simulink model "Waehrungsmodelle"  (R2014a)
settings: Solver=ode1  StartTime=0.0  StopTime=100  FixedStep=1  MaxStep=1  MinStep=1  RelTol=1e-3
(part 1 of 18)
settings Model: Creator=christoph  LastModifiedBy=christoph

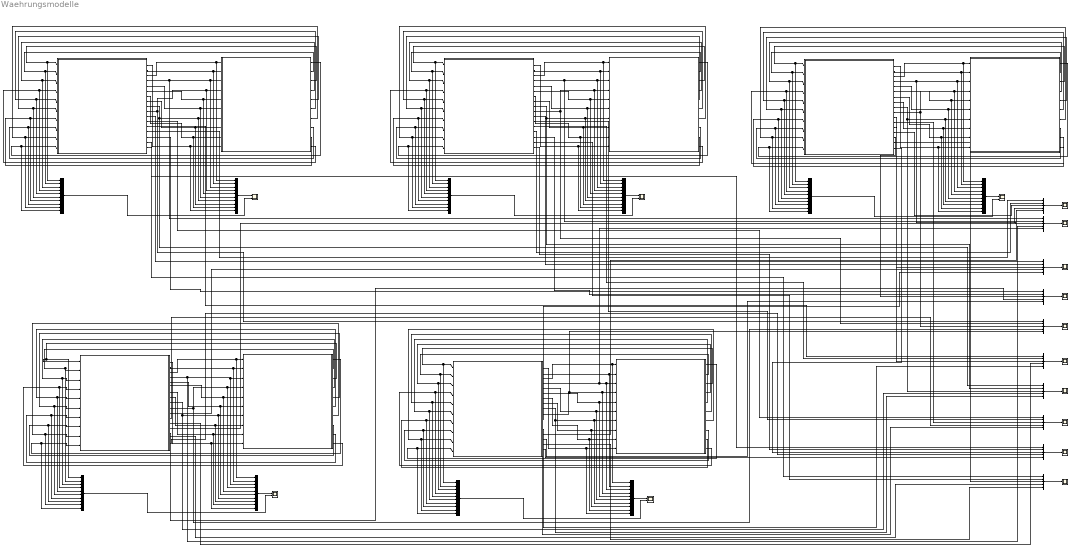
== system Waehrungsmodelle ==
  note: Ungedecktes Währungsmodell
  note: Freies Geld Währungsmodell
  note: Fliessendes Geld Währungsmodell
  note: Vollgeld Währungsmodell
  note: Gedecktes Währungsmodell
  Arbeitslohn : Scope
      settings: ShowLegends=on  YMin=0  YMax=70  SaveName=ScopeData25
  Arbeitslosigkeit : Scope
      settings: ShowLegends=on  YMin=-0.1  YMax=1  SaveName=ScopeData22
  Bankenzins : Scope
      settings: ShowLegends=on  YMin=-0.2  YMax=0.6  SaveName=ScopeData20
  Fließendes Währungssystem : Subsystem
  Freies Geld Währungssystem : Subsystem
  Gedecktes Währungssystem : Subsystem
  Gesamtkredite : Scope
      settings: ShowLegends=on  YMin=0  YMax=9000  SaveName=ScopeData23
  Güterpreise : Scope
      settings: TickLabels=on  ShowLegends=on  TimeRange=100  YMin=0  YMax=35  SaveName=ScopeData21
  Inflation (Preisstabilität) : Scope
      settings: ShowLegends=on  YMin=-0.1  YMax=0.2  SaveName=ScopeData18
  Konsum Ausland : Scope
      settings: ShowLegends=on  YMin=-0.1  YMax=0.2  SaveName=ScopeData27
  Konsum Inland : Scope
      settings: ShowLegends=on  YMin=-0.1  YMax=0.2  SaveName=ScopeData26
  Mux{,1..9} (10 alike) : Mux  Inputs=10
  Mux{10..19} (10 alike) : Mux  Inputs=5
  Notenbankgeldmange / Maximale Geldmenge : Scope
      settings: ShowLegends=on  YMin=0  YMax=10000  SaveName=ScopeData19
  Notenbankzins : Scope
      settings: ShowLegends=on  YMin=-0.05  YMax=0.15  SaveName=ScopeData24
  Scope{,1..4} (5 alike) : Scope  NumInputPorts=2
      Scope settings: ShowLegends=on  YMin=-100~-100  YMax=900~900  SaveName=ScopeData8
      Scope1 settings: ShowLegends=on  YMin=-100~-100  YMax=900~900  SaveName=ScopeData15
      Scope2 settings: ShowLegends=on  YMin=-100~-100  YMax=900~900  SaveName=ScopeData13
      Scope3 settings: ShowLegends=on  YMin=-100~-100  YMax=900~900  SaveName=ScopeData16
      Scope4 settings: ShowLegends=on  YMin=-100~-100  YMax=900~900  SaveName=ScopeData17
  Vollgeld Währungssystem : Subsystem
  Währungssystem1 : Subsystem
  Währungssystem2 : Subsystem
  Währungssystem3 : Subsystem
  Währungssystem4 : Subsystem
  Währungssystem5 : Subsystem
  Währungssystem6 : Subsystem
  wires:
  Währungssystem1/2(Kreditbedarf Ausland Unternehmen) -> Währungssystem2/2(Kreditbedarf der Unternehmen im Ausland), Mux/2
  Währungssystem1/3(Kreditbedarf Ausland Haushalte) -> Währungssystem2/1(Kreditbedarf der Haushalte im Ausland), Mux/1
  Währungssystem1/1(Güterangebot an  Ausland) -> Währungssystem2/10(Güterangebot vom  Ausland), Mux/10
  Währungssystem1/5(Bank: Kreditrückzahlung der Unternemen Ausland) -> Währungssystem2/6(Kreditrückzahlung der Unternehmen Ausland), Mux/6
  Währungssystem1/6("Bank: Kreditvergabe der Unternemen Ausland ") -> Währungssystem2/5(Neue Kreditvergabe der Unternehmen Ausland), Mux/5
  Währungssystem1/7(Bank: Kreditrückzahlung der Haushalte Ausland) -> Währungssystem2/9(Kreditrückzahlung der Haushalte Ausland), Mux/9
  Währungssystem1/8("Bank: Kreditvergabe der Haushalte Ausland ") -> Währungssystem2/8(Neue Kreditvergabe der Haushalte Ausland), Mux/8
  Währungssystem2/1(Güterangebot an  Ausland) -> Mux1/10, Währungssystem1/10(Güterangebot vom  Ausland)
  Währungssystem2/2(Kreditbedarf Ausland Unternehmen) -> Mux1/2, Währungssystem1/2(Kreditbedarf der Unternehmen im Ausland)
  Währungssystem2/3(Kreditbedarf Ausland Haushalte) -> Mux1/1, Währungssystem1/1(Kreditbedarf der Haushalte im Ausland)
  Währungssystem2/4(Güterkonsum vom Ausland) -> Mux1/3, Währungssystem1/3(Güterkonsum Ausland)
  Währungssystem2/5(Bank: Kreditrückzahlung der Unternemen Ausland) -> Mux1/6, Währungssystem1/6(Kreditrückzahlung der Unternehmen Ausland)
  Währungssystem2/6("Bank: Kreditvergabe der Unternemen Ausland ") -> Mux1/5, Währungssystem1/5(Neue Kreditvergabe der Unternehmen Ausland)
  Währungssystem2/7(Bank: Kreditrückzahlung der Haushalte Ausland) -> Mux1/9, Währungssystem1/9(Kreditrückzahlung der Haushalte Ausland)
  Währungssystem2/8("Bank: Kreditvergabe der Haushalte Ausland ") -> Mux1/8, Währungssystem1/8(Neue Kreditvergabe der Haushalte Ausland)
  Währungssystem2/9(Güterpreis) -> Mux1/7, Währungssystem1/7(Güterpreis Ausland)
  Währungssystem2/10(Bankenzinssatz) -> Mux1/4, Währungssystem1/4(Zinssatz Ausland)
  Mux/1 -> Scope/1
  Mux1/1 -> Scope/2
  Freies Geld Währungssystem/2(Kreditbedarf Ausland Unternehmen) -> Währungssystem4/2(Kreditbedarf der Unternehmen im Ausland), Mux2/2
  Freies Geld Währungssystem/3(Kreditbedarf Ausland Haushalte) -> Währungssystem4/1(Kreditbedarf der Haushalte im Ausland), Mux2/1
  Freies Geld Währungssystem/4(Güterkonsum vom Ausland) -> Mux19/4, Währungssystem4/3(Güterkonsum Ausland), Mux2/3
  Freies Geld Währungssystem/1(Güterangebot an  Ausland) -> Währungssystem4/10(Güterangebot vom  Ausland), Mux2/10
  Freies Geld Währungssystem/5(Bank: Kreditrückzahlung der Unternemen Ausland) -> Währungssystem4/6(Kreditrückzahlung der Unternehmen Ausland), Mux2/6
  Freies Geld Währungssystem/6("Bank: Kreditvergabe der Unternemen Ausland ") -> Währungssystem4/5(Neue Kreditvergabe der Unternehmen Ausland), Mux2/5
  Freies Geld Währungssystem/7(Bank: Kreditrückzahlung der Haushalte Ausland) -> Währungssystem4/9(Kreditrückzahlung der Haushalte Ausland), Mux2/9
  Freies Geld Währungssystem/8("Bank: Kreditvergabe der Haushalte Ausland ") -> Währungssystem4/8(Neue Kreditvergabe der Haushalte Ausland), Mux2/8
  Währungssystem4/1(Güterangebot an  Ausland) -> Mux3/10, Freies Geld Währungssystem/10(Güterangebot vom  Ausland)
  Währungssystem4/2(Kreditbedarf Ausland Unternehmen) -> Mux3/2, Freies Geld Währungssystem/2(Kreditbedarf der Unternehmen im Ausland)
  Währungssystem4/3(Kreditbedarf Ausland Haushalte) -> Mux3/1, Freies Geld Währungssystem/1(Kreditbedarf der Haushalte im Ausland)
  Währungssystem4/4(Güterkonsum vom Ausland) -> Mux3/3, Freies Geld Währungssystem/3(Güterkonsum Ausland)
  Währungssystem4/5(Bank: Kreditrückzahlung der Unternemen Ausland) -> Mux3/6, Freies Geld Währungssystem/6(Kreditrückzahlung der Unternehmen Ausland)
  Währungssystem4/6("Bank: Kreditvergabe der Unternemen Ausland ") -> Mux3/5, Freies Geld Währungssystem/5(Neue Kreditvergabe der Unternehmen Ausland)
  Währungssystem4/7(Bank: Kreditrückzahlung der Haushalte Ausland) -> Mux3/9, Freies Geld Währungssystem/9(Kreditrückzahlung der Haushalte Ausland)
  Währungssystem4/8("Bank: Kreditvergabe der Haushalte Ausland ") -> Mux3/8, Freies Geld Währungssystem/8(Neue Kreditvergabe der Haushalte Ausland)
  Währungssystem4/9(Güterpreis) -> Mux3/7, Freies Geld Währungssystem/7(Güterpreis Ausland)
  Währungssystem4/10(Bankenzinssatz) -> Mux3/4, Freies Geld Währungssystem/4(Zinssatz Ausland)
  Mux2/1 -> Scope1/1
  Mux3/1 -> Scope1/2
  Fließendes Währungssystem/2(Kreditbedarf Ausland Unternehmen) -> Währungssystem5/2(Kreditbedarf der Unternehmen im Ausland), Mux4/2
  Fließendes Währungssystem/3(Kreditbedarf Ausland Haushalte) -> Währungssystem5/1(Kreditbedarf der Haushalte im Ausland), Mux4/1
  Fließendes Währungssystem/4(Güterkonsum vom Ausland) -> Mux19/5, Währungssystem5/3(Güterkonsum Ausland), Mux4/3
  Fließendes Währungssystem/1(Güterangebot an  Ausland) -> Währungssystem5/10(Güterangebot vom  Ausland), Mux4/10
  Fließendes Währungssystem/5(Bank: Kreditrückzahlung der Unternemen Ausland) -> Währungssystem5/6(Kreditrückzahlung der Unternehmen Ausland), Mux4/6
  Fließendes Währungssystem/6("Bank: Kreditvergabe der Unternemen Ausland ") -> Währungssystem5/5(Neue Kreditvergabe der Unternehmen Ausland), Mux4/5
  Fließendes Währungssystem/7(Bank: Kreditrückzahlung der Haushalte Ausland) -> Währungssystem5/9(Kreditrückzahlung der Haushalte Ausland), Mux4/9
  Fließendes Währungssystem/8("Bank: Kreditvergabe der Haushalte Ausland ") -> Währungssystem5/8(Neue Kreditvergabe der Haushalte Ausland), Mux4/8
  Währungssystem5/1(Güterangebot an  Ausland) -> Mux5/10, Fließendes Währungssystem/10(Güterangebot vom  Ausland)
  Währungssystem5/2(Kreditbedarf Ausland Unternehmen) -> Mux5/2, Fließendes Währungssystem/2(Kreditbedarf der Unternehmen im Ausland)
  Währungssystem5/3(Kreditbedarf Ausland Haushalte) -> Mux5/1, Fließendes Währungssystem/1(Kreditbedarf der Haushalte im Ausland)
  Währungssystem5/4(Güterkonsum vom Ausland) -> Mux5/3, Fließendes Währungssystem/3(Güterkonsum Ausland)
  Währungssystem5/5(Bank: Kreditrückzahlung der Unternemen Ausland) -> Mux5/6, Fließendes Währungssystem/6(Kreditrückzahlung der Unternehmen Ausland)
  Währungssystem5/6("Bank: Kreditvergabe der Unternemen Ausland ") -> Mux5/5, Fließendes Währungssystem/5(Neue Kreditvergabe der Unternehmen Ausland)
  Währungssystem5/7(Bank: Kreditrückzahlung der Haushalte Ausland) -> Mux5/9, Fließendes Währungssystem/9(Kreditrückzahlung der Haushalte Ausland)
  Währungssystem5/8("Bank: Kreditvergabe der Haushalte Ausland ") -> Mux5/8, Fließendes Währungssystem/8(Neue Kreditvergabe der Haushalte Ausland)
  Währungssystem5/9(Güterpreis) -> Mux5/7, Fließendes Währungssystem/7(Güterpreis Ausland)
  Währungssystem5/10(Bankenzinssatz) -> Mux5/4, Fließendes Währungssystem/4(Zinssatz Ausland)
  Mux4/1 -> Scope2/1
  Mux5/1 -> Scope2/2
  Vollgeld Währungssystem/2(Kreditbedarf Ausland Unternehmen) -> Währungssystem3/2(Kreditbedarf der Unternehmen im Ausland), Mux6/2
  Vollgeld Währungssystem/3(Kreditbedarf Ausland Haushalte) -> Währungssystem3/1(Kreditbedarf der Haushalte im Ausland), Mux6/1
  Vollgeld Währungssystem/4(Güterkonsum vom Ausland) -> Mux19/2, Währungssystem3/3(Güterkonsum Ausland), Mux6/3
  Vollgeld Währungssystem/1(Güterangebot an  Ausland) -> Währungssystem3/10(Güterangebot vom  Ausland), Mux6/10
  Vollgeld Währungssystem/5(Bank: Kreditrückzahlung der Unternemen Ausland) -> Währungssystem3/6(Kreditrückzahlung der Unternehmen Ausland), Mux6/6
  Vollgeld Währungssystem/6("Bank: Kreditvergabe der Unternemen Ausland ") -> Währungssystem3/5(Neue Kreditvergabe der Unternehmen Ausland), Mux6/5
  Vollgeld Währungssystem/7(Bank: Kreditrückzahlung der Haushalte Ausland) -> Währungssystem3/9(Kreditrückzahlung der Haushalte Ausland), Mux6/9
  Vollgeld Währungssystem/8("Bank: Kreditvergabe der Haushalte Ausland ") -> Währungssystem3/8(Neue Kreditvergabe der Haushalte Ausland), Mux6/8
  Vollgeld Währungssystem/9(Güterpreis) -> Währungssystem3/7(Güterpreis Ausland), Mux6/7, Mux14/2
  Währungssystem3/1(Güterangebot an  Ausland) -> Mux7/10, Vollgeld Währungssystem/10(Güterangebot vom  Ausland)
  Währungssystem3/2(Kreditbedarf Ausland Unternehmen) -> Mux7/2, Vollgeld Währungssystem/2(Kreditbedarf der Unternehmen im Ausland)
  Währungssystem3/3(Kreditbedarf Ausland Haushalte) -> Mux7/1, Vollgeld Währungssystem/1(Kreditbedarf der Haushalte im Ausland)
  Währungssystem3/4(Güterkonsum vom Ausland) -> Mux7/3, Vollgeld Währungssystem/3(Güterkonsum Ausland)
  Währungssystem3/5(Bank: Kreditrückzahlung der Unternemen Ausland) -> Mux7/6, Vollgeld Währungssystem/6(Kreditrückzahlung der Unternehmen Ausland)
  Währungssystem3/6("Bank: Kreditvergabe der Unternemen Ausland ") -> Mux7/5, Vollgeld Währungssystem/5(Neue Kreditvergabe der Unternehmen Ausland)
  Währungssystem3/7(Bank: Kreditrückzahlung der Haushalte Ausland) -> Mux7/9, Vollgeld Währungssystem/9(Kreditrückzahlung der Haushalte Ausland)
  Währungssystem3/8("Bank: Kreditvergabe der Haushalte Ausland ") -> Mux7/8, Vollgeld Währungssystem/8(Neue Kreditvergabe der Haushalte Ausland)
  Währungssystem3/9(Güterpreis) -> Mux7/7, Vollgeld Währungssystem/7(Güterpreis Ausland)
  Währungssystem3/10(Bankenzinssatz) -> Mux7/4, Vollgeld Währungssystem/4(Zinssatz Ausland)
  Mux6/1 -> Scope3/1
  Mux7/1 -> Scope3/2
  Gedecktes Währungssystem/2(Kreditbedarf Ausland Unternehmen) -> Währungssystem6/2(Kreditbedarf der Unternehmen im Ausland), Mux8/2
  Gedecktes Währungssystem/3(Kreditbedarf Ausland Haushalte) -> Währungssystem6/1(Kreditbedarf der Haushalte im Ausland), Mux8/1
  Gedecktes Währungssystem/4(Güterkonsum vom Ausland) -> Mux19/3, Währungssystem6/3(Güterkonsum Ausland), Mux8/3
  Gedecktes Währungssystem/1(Güterangebot an  Ausland) -> Währungssystem6/10(Güterangebot vom  Ausland), Mux8/10
  Gedecktes Währungssystem/5(Bank: Kreditrückzahlung der Unternemen Ausland) -> Währungssystem6/6(Kreditrückzahlung der Unternehmen Ausland), Mux8/6
  Gedecktes Währungssystem/6("Bank: Kreditvergabe der Unternemen Ausland ") -> Währungssystem6/5(Neue Kreditvergabe der Unternehmen Ausland), Mux8/5
  Gedecktes Währungssystem/7(Bank: Kreditrückzahlung der Haushalte Ausland) -> Währungssystem6/9(Kreditrückzahlung der Haushalte Ausland), Mux8/9
  Gedecktes Währungssystem/8("Bank: Kreditvergabe der Haushalte Ausland ") -> Währungssystem6/8(Neue Kreditvergabe der Haushalte Ausland), Mux8/8
  Gedecktes Währungssystem/9(Güterpreis) -> Mux14/3, Währungssystem6/7(Güterpreis Ausland), Mux8/7
  Währungssystem6/1(Güterangebot an  Ausland) -> Mux9/10, Gedecktes Währungssystem/10(Güterangebot vom  Ausland)
  Währungssystem6/2(Kreditbedarf Ausland Unternehmen) -> Mux9/2, Gedecktes Währungssystem/2(Kreditbedarf der Unternehmen im Ausland)
  Währungssystem6/3(Kreditbedarf Ausland Haushalte) -> Mux9/1, Gedecktes Währungssystem/1(Kreditbedarf der Haushalte im Ausland)
  Währungssystem6/4(Güterkonsum vom Ausland) -> Mux9/3, Gedecktes Währungssystem/3(Güterkonsum Ausland)
  Währungssystem6/5(Bank: Kreditrückzahlung der Unternemen Ausland) -> Mux9/6, Gedecktes Währungssystem/6(Kreditrückzahlung der Unternehmen Ausland)
  Währungssystem6/6("Bank: Kreditvergabe der Unternemen Ausland ") -> Mux9/5, Gedecktes Währungssystem/5(Neue Kreditvergabe der Unternehmen Ausland)
  Währungssystem6/7(Bank: Kreditrückzahlung der Haushalte Ausland) -> Mux9/9, Gedecktes Währungssystem/9(Kreditrückzahlung der Haushalte Ausland)
  Währungssystem6/8("Bank: Kreditvergabe der Haushalte Ausland ") -> Mux9/8, Gedecktes Währungssystem/8(Neue Kreditvergabe der Haushalte Ausland)
  Währungssystem6/9(Güterpreis) -> Mux9/7, Gedecktes Währungssystem/7(Güterpreis Ausland)
  Währungssystem6/10(Bankenzinssatz) -> Mux9/4, Gedecktes Währungssystem/4(Zinssatz Ausland)
  Mux8/1 -> Scope4/1
  Mux9/1 -> Scope4/2
  Mux10/1 -> Inflation (Preisstabilität)/1
  Gedecktes Währungssystem/11(Inflation) -> Mux10/3
  Vollgeld Währungssystem/11(Inflation) -> Mux10/2
  Währungssystem1/11(Inflation) -> Mux10/1
  Freies Geld Währungssystem/11(Inflation) -> Mux10/4
  Fließendes Währungssystem/11(Inflation) -> Mux10/5
  Mux11/1 -> Notenbankgeldmange / Maximale Geldmenge/1
  Gedecktes Währungssystem/15(Notenbankgeldmenge) -> Mux11/3
  Währungssystem1/15(Notenbankgeldmenge) -> Mux11/1
  Vollgeld Währungssystem/15(Notenbankgeldmenge) -> Mux11/2
  Freies Geld Währungssystem/15(Maximale Geldmenge) -> Mux11/4
  Fließendes Währungssystem/15(Notenbankgeldmenge) -> Mux11/5
  Mux12/1 -> Bankenzins/1
  Mux13/1 -> Notenbankzins/1
  Mux14/1 -> Güterpreise/1
  Mux15/1 -> Arbeitslosigkeit/1
  Mux16/1 -> Gesamtkredite/1
  Währungssystem1/10(Bankenzinssatz) -> Mux12/1, Währungssystem2/4(Zinssatz Ausland), Mux/4
  Vollgeld Währungssystem/10(Bankenzinssatz) -> Währungssystem3/4(Zinssatz Ausland), Mux6/4, Mux12/2
  Gedecktes Währungssystem/10(Bankenzinssatz) -> Mux12/3, Währungssystem6/4(Zinssatz Ausland), Mux8/4
  Freies Geld Währungssystem/10(Bankenzinssatz) -> Mux12/4, Währungssystem4/4(Zinssatz Ausland), Mux2/4
  Fließendes Währungssystem/10(Bankenzinssatz) -> Mux12/5, Währungssystem5/4(Zinssatz Ausland), Mux4/4
  Währungssystem1/13(Notenbankzinsatz) -> Mux13/1
  Vollgeld Währungssystem/13(Notenbankzinsatz) -> Mux13/2
  Gedecktes Währungssystem/13(Notenbankzinsatz) -> Mux13/3
  Freies Geld Währungssystem/13(Notenbankzinsatz) -> Mux13/4
  Fließendes Währungssystem/13(Notenbankzinsatz) -> Mux13/5
  Mux17/1 -> Arbeitslohn/1
  Währungssystem1/9(Güterpreis) -> Währungssystem2/7(Güterpreis Ausland), Mux/7, Mux14/1
  Freies Geld Währungssystem/9(Güterpreis) -> Mux14/4, Währungssystem4/7(Güterpreis Ausland), Mux2/7
  Fließendes Währungssystem/9(Güterpreis) -> Mux14/5, Währungssystem5/7(Güterpreis Ausland), Mux4/7
  Währungssystem1/12(Arbeitslohn) -> Mux17/1
  Vollgeld Währungssystem/12(Arbeitslohn) -> Mux17/2
  Gedecktes Währungssystem/12(Arbeitslohn) -> Mux17/3
  Freies Geld Währungssystem/12(Arbeitslohn) -> Mux17/4
  Fließendes Währungssystem/12(Arbeitslohn) -> Mux17/5
  Währungssystem1/17(Arbeitslosigkeit) -> Mux15/1
  Vollgeld Währungssystem/17(Arbeitslosigkeit) -> Mux15/2
  Gedecktes Währungssystem/17(Arbeitslosigkeit) -> Mux15/3
  Freies Geld Währungssystem/17(Arbeitslosigkeit) -> Mux15/4
  Fließendes Währungssystem/17(Arbeitslosigkeit) -> Mux15/5
  Währungssystem1/16(Gesamtkredite) -> Mux16/1
  Vollgeld Währungssystem/16(Gesamtkredite) -> Mux16/2
  Gedecktes Währungssystem/16(Gesamtkredite) -> Mux16/3
  Freies Geld Währungssystem/16(Gesamtkredite) -> Mux16/4
  Fließendes Währungssystem/16(Gesamtkredite) -> Mux16/5
  Mux18/1 -> Konsum Inland/1
  Mux19/1 -> Konsum Ausland/1
  Währungssystem1/14(Güterkonsum Inland) -> Mux18/1
  Vollgeld Währungssystem/14(Güterkonsum Inland) -> Mux18/2
  Gedecktes Währungssystem/14(Güterkonsum Inland) -> Mux18/3
  Freies Geld Währungssystem/14(Güterkonsum Inland) -> Mux18/4
  Fließendes Währungssystem/14(Güterkonsum Inland) -> Mux18/5
  Währungssystem1/4(Güterkonsum vom Ausland) -> Mux19/1, Währungssystem2/3(Güterkonsum Ausland), Mux/3

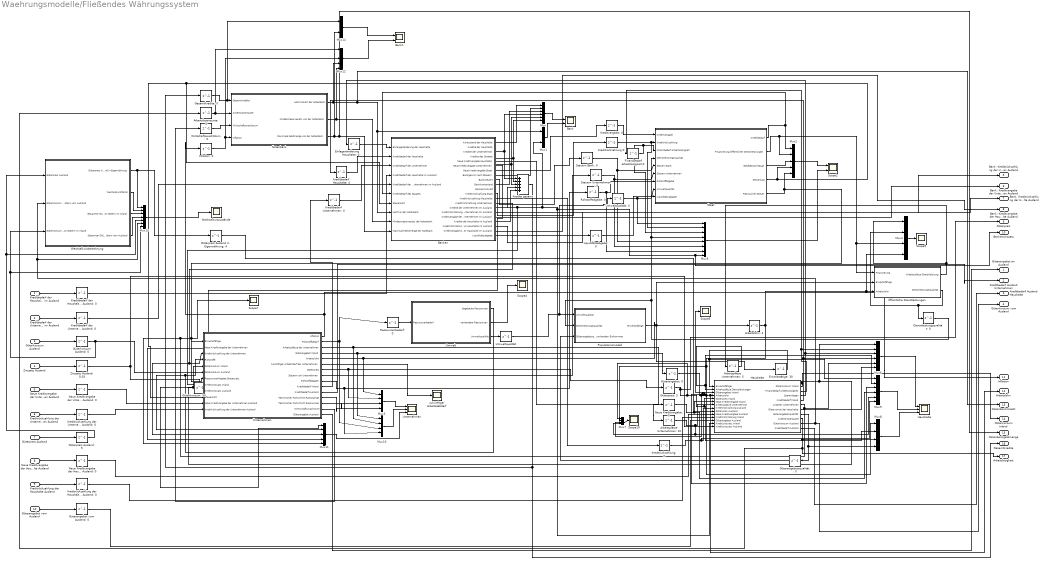
== system Waehrungsmodelle/Fließendes Währungssystem ==
  Kreditbedarf der Haushalte im Ausland : Inport
  Kreditbedarf der Unternehmen im Ausland : Inport  Port=2
  Güterkonsum Ausland : Inport  Port=3
  Zinssatz Ausland : Inport  Port=4
  Neue Kreditvergabe der Unternehmen Ausland : Inport  Port=5
  Kreditrückzahlung der Unternehmen Ausland : Inport  Port=6
  Güterpreis Ausland : Inport  Port=7
  Neue Kreditvergabe der Haushalte Ausland : Inport  Port=8
  Kreditrückzahlung der Haushalte Ausland : Inport  Port=9
  Güterangebot vom  Ausland : Inport  Port=10
  Arbeitslohn: 4 : Delay  DelayLength=1  InitialCondition=4
  Arbeitslosenquote: 0 : Delay  DelayLength=1  InitialCondition=0
  "Arbeitsplätze Unternehmen: 10 " : Delay  DelayLength=1  InitialCondition=10
  Arbeitsplätze Unternehmen: 5 : Delay  DelayLength=1  InitialCondition=5
  Bank : Scope  NumInputPorts=2
      settings: ShowLegends=on  TimeRange=20  YMin=-500~0  YMax=500~0.1
  Bank1 : Scope  NumInputPorts=2
      settings: ShowLegends=on  TimeRange=20  YMin=-500~-0.5  YMax=10000~0.5  SaveName=ScopeData3
  Banken : Subsystem
  Dienstleistungsqualität: 0 : Delay  DelayLength=1  InitialCondition=0
  Einlagenänderung Haushalte: 0 : Delay  DelayLength=1  InitialCondition=0
  Erwerbstätige: 30 : Delay  DelayLength=1  InitialCondition=30
  Finanzbedarf Arbeitslosigkeit:0 : Delay  DelayLength=1  InitialCondition=0
  Gesamtkredite: 0 : Delay  DelayLength=1  InitialCondition=0
  Güterangebot vom  Ausland: 0 : Delay  DelayLength=1  InitialCondition=0
  Güterangebot: 0 : Delay  DelayLength=1  InitialCondition=0
  Güterangebotsqualität: 0 : Delay  DelayLength=1  InitialCondition=0
  Güterkonsum Ausland: 0 : Delay  DelayLength=1  InitialCondition=0
  Güterkonsum: 50 : Delay  DelayLength=1  InitialCondition=50
  Güterpreis Ausland in Eigenwährung: 4 : Delay  DelayLength=1  InitialCondition=4
  Güterpreis Ausland: 5 : Delay  DelayLength=1  InitialCondition=5
  Güterpreis: 3 : Delay  DelayLength=1  InitialCondition=3
  Haushalte : Subsystem
  "Haushalte " : Scope  NumInputPorts=3
      settings: TickLabels=on  ShowLegends=on  TimeRange=100  YMin=-50~0~0  YMax=150~100~1
  Inflation: 0 : Delay  DelayLength=1  InitialCondition=0
  Kreditbedarf Haushalte: 0 : Delay  DelayLength=1  InitialCondition=0
  Kreditbedarf Unternehmen: 0 : Delay  DelayLength=1  InitialCondition=0
  Kreditbedarf der Haushalte im Ausland: 0 : Delay  DelayLength=1  InitialCondition=0
  Kreditbedarf der Unternehmen im Ausland: 0 : Delay  DelayLength=1  InitialCondition=0
  Kredite gesamt : Sum  Inputs=+++++
  Kreditrückzahlung der Haushalte Ausland: 0 : Delay  DelayLength=1  InitialCondition=0
  Kreditrückzahlung der Unternehmen Ausland: 0 : Delay  DelayLength=1  InitialCondition=0
  Kreditrückzahlung: 0 : Delay  DelayLength=1  InitialCondition=0
  Kreditrückzahlung:0 : Delay  DelayLength=1  InitialCondition=0
  Kreditvergabe: 0 : Delay  DelayLength=1  InitialCondition=0
  Liquiditätsabgabe: 0 : Delay  DelayLength=1  InitialCondition=0
  Mux : Mux  Inputs=6
  Mux1 : Mux  Inputs=2
  Mux{3..4,7..8,10} (5 alike) : Mux
  Mux11 : Mux  Inputs=5
  Mux12 : Mux  Inputs=5
  Mux13 : Mux  Inputs=7
  Mux14 : Mux  Inputs=2
  Mux2 : Mux  Inputs=5
  Mux5 : Mux  Inputs=8
  Mux6 : Mux  Inputs=6
  Mux9 : Mux  Inputs=6
  Neue Kreditvergabe der Haushalte Ausland: 0 : Delay  DelayLength=1  InitialCondition=0
  Neue Kreditvergabe der Unternehmen Ausland: 0 : Delay  DelayLength=1  InitialCondition=0
  Neue Kreditvergabe: 0 : Delay  DelayLength=1  InitialCondition=0
  Notenbank : Subsystem
  Populationsmodell : Subsystem
  Ressourcenbedarf: 0 : Delay  DelayLength=1  InitialCondition=0
  Rohstoffabgabe: 0 : Delay  DelayLength=1  InitialCondition=0
  Scope{4..5,7,9..10} (5 alike) : Scope
      Scope10 settings: ShowLegends=on  TimeRange=100  YMin=0  YMax=120  SaveName=ScopeData10
      Scope4 settings: SaveName=ScopeData4
      Scope5 settings: TimeRange=10  YMin=0  YMax=10  SaveName=ScopeData5
      Scope7 settings: ShowLegends=on  TimeRange=10  YMin=9  YMax=15  SaveName=ScopeData7
      Scope9 settings: TickLabels=on  ShowLegends=on  TimeRange=100  YMin=0  YMax=40  SaveName=ScopeData9
  Scope2 : Scope  NumInputPorts=2
      settings: ShowLegends=on  TimeRange=100  YMin=-100~0  YMax=300~500  SaveName=ScopeData2
  Staat : Subsystem
  Steuern Bank: 0 : Delay  DelayLength=1  InitialCondition=0
  Steuern Unternehmen: 0 : Delay  DelayLength=1  InitialCondition=0
  Umwelt : Subsystem
  Umweltqualität : Delay  DelayLength=1  InitialCondition=0
  Umweltqualität: 0 : Delay  DelayLength=1  InitialCondition=0
  Unternehmen : Subsystem
  "Unternehmen " : Scope  NumInputPorts=3
      settings: TickLabels=on  ShowLegends=on  TimeRange=100  YMin=2~-5~-5  YMax=50~200~100  SaveName=ScopeData6
  Wechselkursberechnung : Subsystem
  Wechselkurszustände : Scope
      settings: ShowLegends=on  TimeRange=100  YMin=0  YMax=1  SaveName=ScopeData11
  Wirtschaftswachtstum: 0 : Delay  DelayLength=1  InitialCondition=0
  Zinssatz Ausland: 0.03 : Delay  DelayLength=1  InitialCondition=0.03
  zukünftiger Arbeitsdebdarf : Scope
      settings: ShowLegends=on  TimeRange=10  YMin=9  YMax=15  SaveName=ScopeData14
  Öffentliche Dienstleistungen : Subsystem
  Güterangebot an  Ausland : Outport
  Kreditbedarf Ausland Unternehmen : Outport  Port=2
  Kreditbedarf Ausland Haushalte : Outport  Port=3
  Güterkonsum vom Ausland : Outport  Port=4
  Bank: Kreditrückzahlung der Unternemen Ausland : Outport  Port=5
  "Bank: Kreditvergabe der Unternemen Ausland " : Outport  Port=6
  Bank: Kreditrückzahlung der Haushalte Ausland : Outport  Port=7
  "Bank: Kreditvergabe der Haushalte Ausland " : Outport  Port=8
  Güterpreis : Outport  Port=9
  Bankenzinssatz : Outport  Port=10
  Inflation : Outport  Port=11
  Arbeitslohn : Outport  Port=12
  Notenbankzinsatz : Outport  Port=13
  Güterkonsum Inland : Outport  Port=14
  Notenbankgeldmenge : Outport  Port=15
  Gesamtkredite : Outport  Port=16
  Arbeitslosigkeit : Outport  Port=17
  wires:
  Öffentliche Dienstleistungen/1(Arbeitsplätze Dienstleistung) -> Arbeitsplätze Unternehmen: 5/1, Mux4/1
  Staat/4(Steuersatz) -> Mux2/4, Banken/7(Steuersatz), Unternehmen/10(Steuersatz)
  Umwelt/3(Umweltqualität) -> Umweltqualität/1
  Staat/5(Ressourcen Steuer) -> Unternehmen/7(RessourcenAbgabe Steuersatz), Mux2/5
  Populationsmodell/1(Erwerbsfähige) -> Erwerbstätige: 30/1, Öffentliche Dienstleistungen/2(Erwerbsfähige)
  Unternehmen/7(Güterpreis) -> Mux3/2, Güterpreis: 3/1
  Unternehmen/5(Arbeitslohn) -> Mux3/1, Arbeitslohn: 4/1
  Unternehmen/4(Güterangebot Inland) -> Mux10/1, Güterangebot: 0/1
  Unternehmen/3(Arbeitsplätze der Unternehmen) -> Mux10/2, "Arbeitsplätze Unternehmen: 10 "/1
  Umwelt/1(abgebaute Ressourcen) -> Unternehmen/4(Rohstoffe), Mux11/2
  Haushalte/1(Güterkonsum Inland) -> Güterkonsum Inland/1, Mux6/1, Güterkonsum: 50/1
  Haushalte/7(Güterangebotsqualität) -> Mux8/4, Güterangebotsqualität: 0/1
  Staat/2(Finanzierung Öffentlicher Dienstleistungen) -> Mux2/2, Öffentliche Dienstleistungen/1(Finanzierung), Mux4/3
  Haushalte/5(Arbeiter Unternehmen) -> Mux6/5, Scope7/1, Unternehmen/1(Erwerbsfähige), Mux11/5
  Haushalte/2(Finanzbedarf Arbeitslosigkeit) -> Finanzbedarf Arbeitslosigkeit:0/1, Mux6/2
  Unternehmen/8(Steuern von Unternehmen) -> Steuern Unternehmen: 0/1
  Unternehmen/9(Rohstoffabgabe) -> Mux10/4, Rohstoffabgabe: 0/1
  Haushalte/8(Arbeitslosenquote) -> Arbeitslosigkeit/1, Arbeitslosenquote: 0/1, Mux8/3
  Unternehmen/1(Inflation) -> Inflation/1, Inflation: 0/1
  Unternehmen/14(Wirtschaftswachstum) -> Wirtschaftswachtstum: 0/1
  Notenbank/1(Leitzinssatz der Notenbank) -> Mux12/4, Notenbankzinsatz/1, Mux1/1, Banken/8(Leitzins der Notenbank)
  Notenbank/2(Mindestreservesatz von der Notenbank) -> Mux12/5, Banken/9(Mindestreservesatz der Notenbank)
  Notenbank/3(Maximale Geldmenge von der Notenbank) -> Notenbankgeldmenge/1, Banken/10(Maximale Geldmenge der Notebank), Mux14/2
  Banken/2(Kredite der Haushalte) -> Mux/4, Kredite gesamt/1
  Banken/3(Kredite der Unternehmen) -> Mux/6, Kredite gesamt/2
  Banken/4(Kredite des Staates) -> Mux/5, Kredite gesamt/3
  Banken/9(Banksteuern) -> Steuern Bank: 0/1
  Banken/7(Neue Kreditvergabe Staat) -> Kreditvergabe: 0/1
  Banken/12(Kreditrückzahlung Staat) -> Kreditrückzahlung:0/1
  Banken/13(Kreditrückzahlung Haushalte) -> Kreditrückzahlung: 0/1
  Banken/5(Neue Kreditvergabe Haushalte) -> Neue Kreditvergabe: 0/1
  Haushalte/3(Spareinlagen) -> Einlagenänderung Haushalte: 0/1, Mux6/3
  Haushalte/4(Kreditbedarf Inland) -> Kreditbedarf Haushalte: 0/1, Mux6/4
  Unternehmen/10(Kreditbedarf Inland) -> Kreditbedarf Unternehmen: 0/1
  Staat/1(Kreditbedarf) -> Banken/6(Kreditbedarf des Staates), Mux2/1
  Banken/6(Neue Kreditvergabe Unternehmen) -> Mux11/4, Unternehmen/2(Neue Kreditvergabe der Unternehmen)
  Banken/14(Kreditrückzahlung Unternehmen) -> Unternehmen/3(Kreditrückzahlung der Unternehmen), Mux11/3
  Banken/1(Kontostand der Haushalte) -> Mux/1
  Banken/8(Bankgewinn nach Steuern) -> Mux/2
  Banken/10(Bankkontostand) -> Mux/3
  Banken/11(Bankenzinssatz) -> Haushalte/13(Kreditzinssatz Inland), Bankenzinssatz/1, Mux5/8, Mux1/2, Unternehmen/8(Kreditzinssatz Inland)
  Unternehmen/13(Technischer Fortschritt Ressourcen) -> Mux3/3
  Unternehmen/12(Technischer Fortschritt Rationalität) -> Mux3/4
  Umwelt/2(verhandene Ressourcen) -> Scope4/1
  Kredite gesamt/1 -> Gesamtkredite/1, Gesamtkredite: 0/1
  Gesamtkredite: 0/1 -> Mux14/1, Notenbank/1(Gesamtkredite)
  Wirtschaftswachtstum: 0/1 -> Notenbank/3(Wirtschaftswachtsum)
  Inflation: 0/1 -> Mux12/3, Notenbank/4(Inflation)
  Ressourcenbedarf: 0/1 -> Umwelt/1(Ressourcenbedarf)
  Unternehmen/2(Rohstoffbedarf) -> Ressourcenbedarf: 0/1, Mux10/3
  Umweltqualität: 0/1 -> Mux5/1, Staat/8(Umweltqualität)
  Rohstoffabgabe: 0/1 -> Mux5/7, Staat/7(Rohstoffabgabe)
  Dienstleistungsqualität: 0/1 -> Populationsmodell/2(Dienstleistungsqualität), Staat/4(Dienstleistungsqualität), Mux5/4
  Steuern Unternehmen: 0/1 -> Mux5/6, Staat/6(Steuern Unternehmen)
  Steuern Bank: 0/1 -> Staat/5(Steuern Bank), Mux5/5
  Finanzbedarf Arbeitslosigkeit:0/1 -> Mux5/3, Staat/3(Finanzbedarf Arbeitslosigkeit)
  Kreditrückzahlung:0/1 -> Staat/2(Kreditrückzahlung), Mux5/2
  Kreditvergabe: 0/1 -> Staat/1(Kreditvergabe)
  Umweltqualität/1 -> Umweltqualität: 0/1, Populationsmodell/1(Umweltqualität)
  Öffentliche Dienstleistungen/2(Dienstleistungsqualität) -> Dienstleistungsqualität: 0/1, Mux4/2
  Güterangebotsqualität: 0/1 -> Populationsmodell/3(Güterangebotsqualität bei vorhandem Einkommen)
  "Arbeitsplätze Unternehmen: 10 "/1 -> Mux9/5, Mux7/4, Haushalte/7(Arbeitsplätze Unternehmen)
  Kreditrückzahlung: 0/1 -> Mux9/6, Haushalte/8(Kreditrückzahlung Ausland)
  Neue Kreditvergabe: 0/1 -> Mux9/4, Haushalte/6(Neue Kreditvergabe Inland)
  Arbeitslohn: 4/1 -> Mux8/1, Arbeitslohn/1, Haushalte/4(Arbeitslohn), Mux7/2, Mux4/4, Öffentliche Dienstleistungen/3(Arbeitslohn)
  Güterangebot: 0/1 -> Mux7/3, Mux9/3, Haushalte/3(Güterangebot Inland), Scope5/1
  Arbeitsplätze Unternehmen: 5/1 -> Haushalte/2(Arbeitsplätze Dienstleistungen), Mux9/2
  Erwerbstätige: 30/1 -> Haushalte/1(Erwerbsfähige), Mux9/1
  Güterkonsum: 50/1 -> Unternehmen/5(Güterkonsum Inland), Mux11/1
  Mux4/1 -> Scope9/1
  Staat/3(Geldbestand Staat) -> Mux2/3
  Mux2/1 -> Scope2/1
  Mux5/1 -> Scope2/2
  Mux/1 -> Bank/1
  Mux7/1 -> Scope10/1
  Mux1/1 -> Bank/2
  Mux6/1 -> "Haushalte "/1
  Mux8/1 -> "Haushalte "/3
  Haushalte/6(Gütervorrat der Haushalte) -> Mux6/6
  Mux9/1 -> "Haushalte "/2
  Mux3/1 -> "Unternehmen "/1
  Mux10/1 -> "Unternehmen "/2
  Mux11/1 -> "Unternehmen "/3
  Güterkonsum Ausland/1 -> Güterkonsum Ausland: 0/1
  Zinssatz Ausland: 0.03/1 -> Haushalte/14(Kreditzinssatz Ausland), Unternehmen/9(Kreditzinssatz Ausland)
  Unternehmen/15(Güterangebot Ausland) -> Güterangebot an  Ausland/1
  Kreditbedarf Haushalte: 0/1 -> Banken/2(Kreditbedarf der Haushalte)
  Kreditbedarf Unternehmen: 0/1 -> Banken/3(Kreditbedarf der Unternehmen)
  Einlagenänderung Haushalte: 0/1 -> Banken/1(Einlangenänderung der Haushalte)
  Kreditbedarf der Haushalte im Ausland: 0/1 -> Banken/4(Kreditbedarf der Haushalte im Ausland)
  Kreditbedarf der Unternehmen im Ausland: 0/1 -> Banken/5(Kreditbedarf der Unternehmen im Ausland)
  Neue Kreditvergabe der Unternehmen Ausland/1 -> Neue Kreditvergabe der Unternehmen Ausland: 0/1
  Kreditrückzahlung der Unternehmen Ausland/1 -> Kreditrückzahlung der Unternehmen Ausland: 0/1
  Banken/16(Kreditrückzahlung der Unternehmen im Ausland) -> Bank: Kreditrückzahlung der Unternemen Ausland/1
  Banken/18(Kredite der Haushalte im Ausland) -> Kredite gesamt/5
  Banken/15(Kredite der Unternehmen im Ausland) -> Kredite gesamt/4
  Neue Kreditvergabe der Haushalte Ausland/1 -> Neue Kreditvergabe der Haushalte Ausland: 0/1
  Unternehmen/11(Kreditbedarf Ausland) -> Kreditbedarf Ausland Unternehmen/1
  Kreditrückzahlung der Haushalte Ausland/1 -> Kreditrückzahlung der Haushalte Ausland: 0/1
  Haushalte/10(Kreditbedarf Ausland) -> Kreditbedarf Ausland Haushalte/1
  Banken/20(Kreditvergabe der Haushalte im Ausland) -> "Bank: Kreditvergabe der Haushalte Ausland "/1
  Güterangebot vom  Ausland/1 -> Güterangebot vom  Ausland: 0/1
  Unternehmen/6(zukünftiger Arbeitsdarf der Unternehmen) -> zukünftiger Arbeitsdebdarf/1
  Banken/17(Kreditvergabe der Unternehmen im Ausland) -> "Bank: Kreditvergabe der Unternemen Ausland "/1
  Banken/19(Kreditrückzahlung der Haushalte im Ausland) -> Bank: Kreditrückzahlung der Haushalte Ausland/1
  Güterpreis: 3/1 -> Güterpreis/1, Mux7/1, Mux8/2, Haushalte/5(Güterpreis Inland)
  Kreditbedarf der Haushalte im Ausland/1 -> Kreditbedarf der Haushalte im Ausland: 0/1
  Kreditbedarf der Unternehmen im Ausland/1 -> Kreditbedarf der Unternehmen im Ausland: 0/1
  Güterkonsum Ausland: 0/1 -> Mux13/7, Wechselkursberechnung/3(Güterkonsum im Ausland von Gütern im Inland), Unternehmen/6(Güterkonsum Ausland)
  Zinssatz Ausland/1 -> Zinssatz Ausland: 0.03/1
  Neue Kreditvergabe der Unternehmen Ausland: 0/1 -> Unternehmen/11(Neue Kreditvergabe der Unternehmen Ausland)
  Kreditrückzahlung der Unternehmen Ausland: 0/1 -> Unternehmen/12(Kreditrückzahlung der Unternehmen Ausland)
  Güterpreis Ausland: 5/1 -> Mux13/5, Wechselkursberechnung/1(Güterpreis Ausland)
  Neue Kreditvergabe der Haushalte Ausland: 0/1 -> Haushalte/10(Neue Kreditvergabe Ausland)
  Kreditrückzahlung der Haushalte Ausland: 0/1 -> Haushalte/11(Kreditrückzahlung Inland)
  Güterangebot vom  Ausland: 0/1 -> Haushalte/12(Güterangebot Ausland)
  Mux14/1 -> Bank1/1
  Mux12/1 -> Bank1/2
  Arbeitslosenquote: 0/1 -> Notenbank/2(Arbeitslosenquote), Mux12/1
  Güterpreis Ausland/1 -> Güterpreis Ausland: 5/1
  Wechselkursberechnung/1(Güterpreis Ausland in Eigenwährung) -> Güterpreis Ausland in Eigenwährung: 4/1, Mux13/1
  Haushalte/9(Güterkonsum Ausland) -> Mux13/6, Wechselkursberechnung/2(Güterkonsum im Inland von Gütern vom Ausland), Güterkonsum vom Ausland/1
  Güterpreis Ausland in Eigenwährung: 4/1 -> Haushalte/9(Güterpreis Ausland)
  Wechselkursberechnung/3(Gesamter Güterkonsum im Ausland von Gütern im Inland) -> Mux13/3
  Wechselkursberechnung/2(Wechselkursfaktor) -> Mux13/2
  Wechselkursberechnung/4(Gesamter Güterkonsum im Inland von Gütern vom Ausland) -> Mux13/4
  Mux13/1 -> Wechselkurszustände/1
  Banken/21(Liquiditätsabgabe) -> Liquiditätsabgabe: 0/1
  Liquiditätsabgabe: 0/1 -> Staat/9(Liquiditätsabgabe)

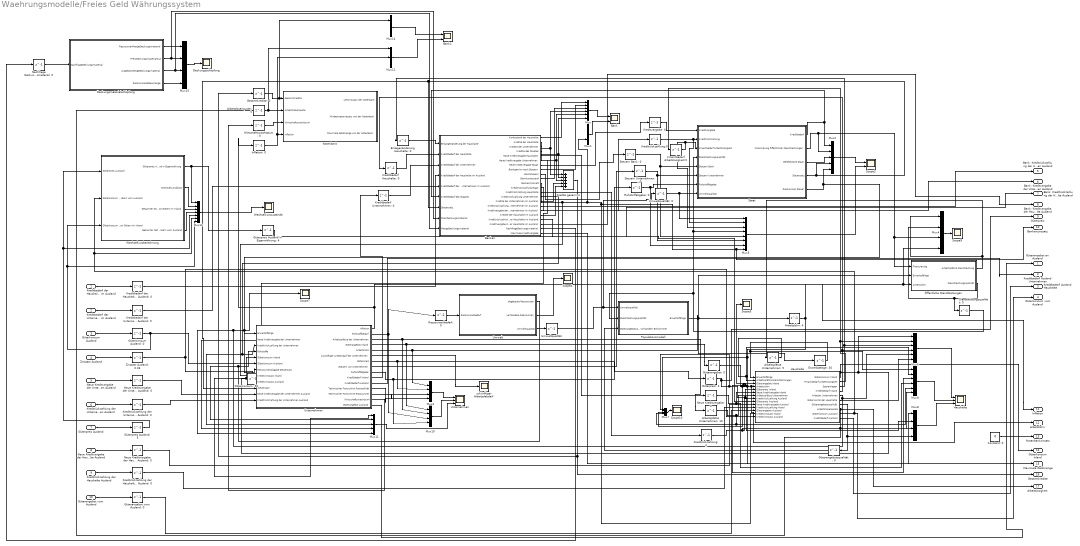
== system Waehrungsmodelle/Freies Geld Währungssystem ==
  Kreditbedarf der Haushalte im Ausland : Inport
  Kreditbedarf der Unternehmen im Ausland : Inport  Port=2
  Güterkonsum Ausland : Inport  Port=3
  Zinssatz Ausland : Inport  Port=4
  Neue Kreditvergabe der Unternehmen Ausland : Inport  Port=5
  Kreditrückzahlung der Unternehmen Ausland : Inport  Port=6
  Güterpreis Ausland : Inport  Port=7
  Neue Kreditvergabe der Haushalte Ausland : Inport  Port=8
  Kreditrückzahlung der Haushalte Ausland : Inport  Port=9
  Güterangebot vom  Ausland : Inport  Port=10
  Arbeitslohn: 4 : Delay  DelayLength=1  InitialCondition=4
  Arbeitslosenquote: 0 : Delay  DelayLength=1  InitialCondition=0
  "Arbeitsplätze Unternehmen: 10 " : Delay  DelayLength=1  InitialCondition=10
  Arbeitsplätze Unternehmen: 5 : Delay  DelayLength=1  InitialCondition=5
  Bank : Scope  NumInputPorts=2
      settings: ShowLegends=on  TimeRange=20  YMin=-500~0  YMax=500~0.5
  Bank1 : Scope  NumInputPorts=2
      settings: ShowLegends=on  TimeRange=20  YMin=-500~-0.5  YMax=10000~0.5  SaveName=ScopeData3
  Banken : Subsystem
  Constant: 0 : Constant  Value=0
  Deckungsmaterialschöpfung : Subsystem
  Deckungsschöpfung : Scope
      settings: ShowLegends=on  TimeRange=100  YMin=-10  YMax=100  SaveName=ScopeData12
  Dienstleistungsqualität: 0 : Delay  DelayLength=1  InitialCondition=0
  Einlagenänderung Haushalte: 0 : Delay  DelayLength=1  InitialCondition=0
  Erwerbstätige: 30 : Delay  DelayLength=1  InitialCondition=30
  Finanzbedarf Arbeitslosigkeit:0 : Delay  DelayLength=1  InitialCondition=0
  Gesamtkredite: 0 : Delay  DelayLength=1  InitialCondition=0
  Güterangebot vom  Ausland: 0 : Delay  DelayLength=1  InitialCondition=0
  Güterangebot: 0 : Delay  DelayLength=1  InitialCondition=0
  Güterangebotsqualität: 0 : Delay  DelayLength=1  InitialCondition=0
  Güterkonsum Ausland: 0 : Delay  DelayLength=1  InitialCondition=0
  Güterkonsum: 50 : Delay  DelayLength=1  InitialCondition=50
  Güterpreis Ausland in Eigenwährung: 4 : Delay  DelayLength=1  InitialCondition=4
  Güterpreis Ausland: 5 : Delay  DelayLength=1  InitialCondition=5
  Güterpreis: 3 : Delay  DelayLength=1  InitialCondition=3
  Haushalte : Subsystem
  "Haushalte " : Scope  NumInputPorts=3
      settings: TickLabels=on  ShowLegends=on  TimeRange=100  YMin=-50~0~0  YMax=150~100~1
  Inflation: 0 : Delay  DelayLength=1  InitialCondition=0
  Kreditbedarf Haushalte: 0 : Delay  DelayLength=1  InitialCondition=0
  Kreditbedarf Unternehmen: 0 : Delay  DelayLength=1  InitialCondition=0
  Kreditbedarf der Haushalte im Ausland: 0 : Delay  DelayLength=1  InitialCondition=0
  Kreditbedarf der Unternehmen im Ausland: 0 : Delay  DelayLength=1  InitialCondition=0
  Kredite gesammt : Sum  Inputs=+++++
  Kreditrückzahlung der Haushalte Ausland: 0 : Delay  DelayLength=1  InitialCondition=0
  Kreditrückzahlung der Unternehmen Ausland: 0 : Delay  DelayLength=1  InitialCondition=0
  Kreditrückzahlung: 0 : Delay  DelayLength=1  InitialCondition=0
  Kreditrückzahlung:0 : Delay  DelayLength=1  InitialCondition=0
  Kreditvergabe: 0 : Delay  DelayLength=1  InitialCondition=0
  Mux : Mux  Inputs=6
  Mux1 : Mux  Inputs=2
  Mux{3..4,7..8,10,15} (6 alike) : Mux
  Mux11 : Mux  Inputs=5
  Mux12 : Mux  Inputs=5
  Mux13 : Mux  Inputs=7
  Mux14 : Mux  Inputs=2
  Mux2 : Mux  Inputs=5
  Mux5 : Mux  Inputs=8
  Mux6 : Mux  Inputs=6
  Mux9 : Mux  Inputs=6
  Nachfrage Deckungsmaterial: 0 : Delay  DelayLength=1  InitialCondition=0
  Neue Kreditvergabe der Haushalte Ausland: 0 : Delay  DelayLength=1  InitialCondition=0
  Neue Kreditvergabe der Unternehmen Ausland: 0 : Delay  DelayLength=1  InitialCondition=0
  Neue Kreditvergabe: 0 : Delay  DelayLength=1  InitialCondition=0
  Notenbank : Subsystem
  Populationsmodell : Subsystem
  Ressourcenbedarf: 0 : Delay  DelayLength=1  InitialCondition=0
  Rohstoffabgabe: 0 : Delay  DelayLength=1  InitialCondition=0
  Scope{4..5,7,9..10} (5 alike) : Scope
      Scope10 settings: ShowLegends=on  TimeRange=100  YMin=0  YMax=120  SaveName=ScopeData10
      Scope4 settings: SaveName=ScopeData4
      Scope5 settings: TimeRange=10  YMin=0  YMax=10  SaveName=ScopeData5
      Scope7 settings: ShowLegends=on  TimeRange=10  YMin=9  YMax=15  SaveName=ScopeData7
      Scope9 settings: TickLabels=on  ShowLegends=on  TimeRange=100  YMin=0  YMax=40  SaveName=ScopeData9
  Scope2 : Scope  NumInputPorts=2
      settings: ShowLegends=on  TimeRange=100  YMin=-100~0  YMax=300~500  SaveName=ScopeData2
  Staat : Subsystem
  Steuern Bank: 0 : Delay  DelayLength=1  InitialCondition=0
  Steuern Unternehmen: 0 : Delay  DelayLength=1  InitialCondition=0
  Umwelt : Subsystem
  Umweltqualität : Delay  DelayLength=1  InitialCondition=0
  Umweltqualität: 0 : Delay  DelayLength=1  InitialCondition=0
  Unternehmen : Subsystem
  "Unternehmen " : Scope  NumInputPorts=3
      settings: TickLabels=on  ShowLegends=on  TimeRange=100  YMin=2~-5~-5  YMax=50~200~100  SaveName=ScopeData6
  Wechselkursberechnung : Subsystem
  Wechselkurszustände : Scope
      settings: ShowLegends=on  TimeRange=100  YMin=0  YMax=1  SaveName=ScopeData11
  Wirtschaftswachtstum: 0 : Delay  DelayLength=1  InitialCondition=0
  Zinssatz Ausland: 0.03 : Delay  DelayLength=1  InitialCondition=0.03
  zukünftiger Arbeitsdebdarf : Scope
      settings: ShowLegends=on  TimeRange=10  YMin=9  YMax=15  SaveName=ScopeData14
  Öffentliche Dienstleistungen : Subsystem
  Güterangebot an  Ausland : Outport
  Kreditbedarf Ausland Unternehmen : Outport  Port=2
  Kreditbedarf Ausland Haushalte : Outport  Port=3
  Güterkonsum vom Ausland : Outport  Port=4
  Bank: Kreditrückzahlung der Unternemen Ausland : Outport  Port=5
  "Bank: Kreditvergabe der Unternemen Ausland " : Outport  Port=6
  Bank: Kreditrückzahlung der Haushalte Ausland : Outport  Port=7
  "Bank: Kreditvergabe der Haushalte Ausland " : Outport  Port=8
  Güterpreis : Outport  Port=9
  Bankenzinssatz : Outport  Port=10
  Inflation : Outport  Port=11
  Arbeitslohn : Outport  Port=12
  Notenbankzinsatz : Outport  Port=13
  Güterkonsum Inland : Outport  Port=14
  Maximale Geldmenge : Outport  Port=15
  Gesamtkredite : Outport  Port=16
  Arbeitslosigkeit : Outport  Port=17
  wires:
  Öffentliche Dienstleistungen/1(Arbeitsplätze Dienstleistung) -> Arbeitsplätze Unternehmen: 5/1, Mux4/1
  Staat/4(Steuersatz) -> Mux2/4, Unternehmen/10(Steuersatz), Banken/7(Steuersatz)
  Umwelt/3(Umweltqualität) -> Umweltqualität/1
  Staat/5(Ressourcen Steuer) -> Unternehmen/7(RessourcenAbgabe Steuersatz), Mux2/5
  Populationsmodell/1(Erwerbsfähige) -> Erwerbstätige: 30/1, Öffentliche Dienstleistungen/2(Erwerbsfähige)
  Unternehmen/7(Güterpreis) -> Mux3/2, Güterpreis: 3/1
  Unternehmen/5(Arbeitslohn) -> Mux3/1, Arbeitslohn: 4/1
  Unternehmen/4(Güterangebot Inland) -> Mux10/1, Güterangebot: 0/1
  Unternehmen/3(Arbeitsplätze der Unternehmen) -> Mux10/2, "Arbeitsplätze Unternehmen: 10 "/1
  Umwelt/1(abgebaute Ressourcen) -> Unternehmen/4(Rohstoffe), Mux11/2
  Haushalte/1(Güterkonsum Inland) -> Güterkonsum Inland/1, Mux6/1, Güterkonsum: 50/1
  Haushalte/7(Güterangebotsqualität) -> Mux8/4, Güterangebotsqualität: 0/1
  Staat/2(Finanzierung Öffentlicher Dienstleistungen) -> Mux2/2, Öffentliche Dienstleistungen/1(Finanzierung), Mux4/3
  Haushalte/5(Arbeiter Unternehmen) -> Mux6/5, Scope7/1, Unternehmen/1(Erwerbsfähige), Mux11/5
  Haushalte/2(Finanzbedarf Arbeitslosigkeit) -> Finanzbedarf Arbeitslosigkeit:0/1, Mux6/2
  Unternehmen/8(Steuern von Unternehmen) -> Steuern Unternehmen: 0/1
  Unternehmen/9(Rohstoffabgabe) -> Mux10/4, Rohstoffabgabe: 0/1
  Haushalte/8(Arbeitslosenquote) -> Arbeitslosigkeit/1, Arbeitslosenquote: 0/1, Mux8/3
  Unternehmen/1(Inflation) -> Inflation/1, Inflation: 0/1
  Unternehmen/14(Wirtschaftswachstum) -> Wirtschaftswachtstum: 0/1
  Banken/2(Kredite der Haushalte) -> Mux/4, Kredite gesammt/1
  Banken/3(Kredite der Unternehmen) -> Mux/6, Kredite gesammt/2
  Banken/4(Kredite des Staates) -> Mux/5, Kredite gesammt/3
  Banken/9(Banksteuern) -> Steuern Bank: 0/1
  Banken/7(Neue Kreditvergabe Staat) -> Kreditvergabe: 0/1
  Banken/12(Kreditrückzahlung Staat) -> Kreditrückzahlung:0/1
  Banken/13(Kreditrückzahlung Haushalte) -> Kreditrückzahlung: 0/1
  Banken/5(Neue Kreditvergabe Haushalte) -> Neue Kreditvergabe: 0/1
  Haushalte/3(Spareinlagen) -> Einlagenänderung Haushalte: 0/1, Mux6/3
  Haushalte/4(Kreditbedarf Inland) -> Kreditbedarf Haushalte: 0/1, Mux6/4
  Unternehmen/10(Kreditbedarf Inland) -> Kreditbedarf Unternehmen: 0/1
  Staat/1(Kreditbedarf) -> Banken/6(Kreditbedarf des Staates), Mux2/1
  Banken/6(Neue Kreditvergabe Unternehmen) -> Mux11/4, Unternehmen/2(Neue Kreditvergabe der Unternehmen)
  Banken/14(Kreditrückzahlung Unternehmen) -> Unternehmen/3(Kreditrückzahlung der Unternehmen), Mux11/3
  Banken/1(Kontostand der Haushalte) -> Mux/1
  Banken/8(Bankgewinn nach Steuern) -> Mux/2
  Banken/10(Bankkontostand) -> Mux/3
  Banken/11(Bankenzinssatz) -> Haushalte/13(Kreditzinssatz Inland), Bankenzinssatz/1, Mux5/8, Mux1/2, Unternehmen/8(Kreditzinssatz Inland)
  Unternehmen/13(Technischer Fortschritt Ressourcen) -> Mux3/3
  Unternehmen/12(Technischer Fortschritt Rationalität) -> Mux3/4
  Umwelt/2(verhandene Ressourcen) -> Scope4/1
  Kredite gesammt/1 -> Gesamtkredite/1, Gesamtkredite: 0/1
  Gesamtkredite: 0/1 -> Mux14/1, Notenbank/1(Gesamtkredite)
  Wirtschaftswachtstum: 0/1 -> Notenbank/3(Wirtschaftswachtsum)
  Inflation: 0/1 -> Mux12/3, Notenbank/4(Inflation)
  Ressourcenbedarf: 0/1 -> Umwelt/1(Ressourcenbedarf)
  Unternehmen/2(Rohstoffbedarf) -> Ressourcenbedarf: 0/1, Mux10/3
  Umweltqualität: 0/1 -> Mux5/1, Staat/8(Umweltqualität)
  Rohstoffabgabe: 0/1 -> Mux5/7, Staat/7(Rohstoffabgabe)
  Dienstleistungsqualität: 0/1 -> Populationsmodell/2(Dienstleistungsqualität), Staat/4(Dienstleistungsqualität), Mux5/4
  Steuern Unternehmen: 0/1 -> Mux5/6, Staat/6(Steuern Unternehmen)
  Steuern Bank: 0/1 -> Staat/5(Steuern Bank), Mux5/5
  Finanzbedarf Arbeitslosigkeit:0/1 -> Mux5/3, Staat/3(Finanzbedarf Arbeitslosigkeit)
  Kreditrückzahlung:0/1 -> Staat/2(Kreditrückzahlung), Mux5/2
  Kreditvergabe: 0/1 -> Staat/1(Kreditvergabe)
  Umweltqualität/1 -> Umweltqualität: 0/1, Populationsmodell/1(Umweltqualität)
  Öffentliche Dienstleistungen/2(Dienstleistungsqualität) -> Dienstleistungsqualität: 0/1, Mux4/2
  Güterangebotsqualität: 0/1 -> Populationsmodell/3(Güterangebotsqualität bei vorhandem Einkommen)
  "Arbeitsplätze Unternehmen: 10 "/1 -> Mux9/5, Mux7/4, Haushalte/7(Arbeitsplätze Unternehmen)
  Kreditrückzahlung: 0/1 -> Mux9/6, Haushalte/8(Kreditrückzahlung Ausland)
  Neue Kreditvergabe: 0/1 -> Mux9/4, Haushalte/6(Neue Kreditvergabe Inland)
  Arbeitslohn: 4/1 -> Mux8/1, Arbeitslohn/1, Haushalte/4(Arbeitslohn), Mux7/2, Mux4/4, Öffentliche Dienstleistungen/3(Arbeitslohn)
  Güterangebot: 0/1 -> Mux7/3, Mux9/3, Haushalte/3(Güterangebot Inland), Scope5/1
  Arbeitsplätze Unternehmen: 5/1 -> Haushalte/2(Arbeitsplätze Dienstleistungen), Mux9/2
  Erwerbstätige: 30/1 -> Haushalte/1(Erwerbsfähige), Mux9/1
  Güterkonsum: 50/1 -> Unternehmen/5(Güterkonsum Inland), Mux11/1
  Mux4/1 -> Scope9/1
  Staat/3(Geldbestand Staat) -> Mux2/3
  Mux2/1 -> Scope2/1
  Mux5/1 -> Scope2/2
  Mux/1 -> Bank/1
  Mux7/1 -> Scope10/1
  Mux1/1 -> Bank/2
  Mux6/1 -> "Haushalte "/1
  Mux8/1 -> "Haushalte "/3
  Haushalte/6(Gütervorrat der Haushalte) -> Mux6/6
  Mux9/1 -> "Haushalte "/2
  Mux3/1 -> "Unternehmen "/1
  Mux10/1 -> "Unternehmen "/2
  Mux11/1 -> "Unternehmen "/3
  Güterkonsum Ausland/1 -> Güterkonsum Ausland: 0/1
  Zinssatz Ausland: 0.03/1 -> Haushalte/14(Kreditzinssatz Ausland), Unternehmen/9(Kreditzinssatz Ausland)
  Unternehmen/15(Güterangebot Ausland) -> Güterangebot an  Ausland/1
  Kreditbedarf Haushalte: 0/1 -> Banken/2(Kreditbedarf der Haushalte)
  Kreditbedarf Unternehmen: 0/1 -> Banken/3(Kreditbedarf der Unternehmen)
  Einlagenänderung Haushalte: 0/1 -> Banken/1(Einlangenänderung der Haushalte)
  Kreditbedarf der Haushalte im Ausland: 0/1 -> Banken/4(Kreditbedarf der Haushalte im Ausland)
  Kreditbedarf der Unternehmen im Ausland: 0/1 -> Banken/5(Kreditbedarf der Unternehmen im Ausland)
  Neue Kreditvergabe der Unternehmen Ausland/1 -> Neue Kreditvergabe der Unternehmen Ausland: 0/1
  Kreditrückzahlung der Unternehmen Ausland/1 -> Kreditrückzahlung der Unternehmen Ausland: 0/1
  Banken/16(Kreditrückzahlung der Unternehmen im Ausland) -> Bank: Kreditrückzahlung der Unternemen Ausland/1
  Banken/18(Kredite der Haushalte im Ausland) -> Kredite gesammt/5
  Banken/15(Kredite der Unternehmen im Ausland) -> Kredite gesammt/4
  Neue Kreditvergabe der Haushalte Ausland/1 -> Neue Kreditvergabe der Haushalte Ausland: 0/1
  Unternehmen/11(Kreditbedarf Ausland) -> Kreditbedarf Ausland Unternehmen/1
  Kreditrückzahlung der Haushalte Ausland/1 -> Kreditrückzahlung der Haushalte Ausland: 0/1
  Haushalte/10(Kreditbedarf Ausland) -> Kreditbedarf Ausland Haushalte/1
  Banken/20(Kreditvergabe der Haushalte im Ausland) -> "Bank: Kreditvergabe der Haushalte Ausland "/1
  Güterangebot vom  Ausland/1 -> Güterangebot vom  Ausland: 0/1
  Unternehmen/6(zukünftiger Arbeitsdarf der Unternehmen) -> zukünftiger Arbeitsdebdarf/1
  Banken/17(Kreditvergabe der Unternehmen im Ausland) -> "Bank: Kreditvergabe der Unternemen Ausland "/1
  Banken/19(Kreditrückzahlung der Haushalte im Ausland) -> Bank: Kreditrückzahlung der Haushalte Ausland/1
  Güterpreis: 3/1 -> Güterpreis/1, Mux7/1, Mux8/2, Haushalte/5(Güterpreis Inland)
  Kreditbedarf der Haushalte im Ausland/1 -> Kreditbedarf der Haushalte im Ausland: 0/1
  Kreditbedarf der Unternehmen im Ausland/1 -> Kreditbedarf der Unternehmen im Ausland: 0/1
  Güterkonsum Ausland: 0/1 -> Mux13/7, Wechselkursberechnung/3(Güterkonsum im Ausland von Gütern im Inland), Unternehmen/6(Güterkonsum Ausland)
  Zinssatz Ausland/1 -> Zinssatz Ausland: 0.03/1
  Neue Kreditvergabe der Unternehmen Ausland: 0/1 -> Unternehmen/11(Neue Kreditvergabe der Unternehmen Ausland)
  Kreditrückzahlung der Unternehmen Ausland: 0/1 -> Unternehmen/12(Kreditrückzahlung der Unternehmen Ausland)
  Güterpreis Ausland: 5/1 -> Mux13/5, Wechselkursberechnung/1(Güterpreis Ausland)
  Neue Kreditvergabe der Haushalte Ausland: 0/1 -> Haushalte/10(Neue Kreditvergabe Ausland)
  Kreditrückzahlung der Haushalte Ausland: 0/1 -> Haushalte/11(Kreditrückzahlung Inland)
  Güterangebot vom  Ausland: 0/1 -> Haushalte/12(Güterangebot Ausland)
  Mux14/1 -> Bank1/1
  Mux12/1 -> Bank1/2
  Arbeitslosenquote: 0/1 -> Notenbank/2(Arbeitslosenquote), Mux12/1
  Güterpreis Ausland/1 -> Güterpreis Ausland: 5/1
  Wechselkursberechnung/1(Güterpreis Ausland in Eigenwährung) -> Güterpreis Ausland in Eigenwährung: 4/1, Mux13/1
  Haushalte/9(Güterkonsum Ausland) -> Mux13/6, Wechselkursberechnung/2(Güterkonsum im Inland von Gütern vom Ausland), Güterkonsum vom Ausland/1
  Güterpreis Ausland in Eigenwährung: 4/1 -> Haushalte/9(Güterpreis Ausland)
  Wechselkursberechnung/3(Gesamter Güterkonsum im Ausland von Gütern im Inland) -> Mux13/3
  Wechselkursberechnung/2(Wechselkursfaktor) -> Mux13/2
  Wechselkursberechnung/4(Gesamter Güterkonsum im Inland von Gütern vom Ausland) -> Mux13/4
  Mux13/1 -> Wechselkurszustände/1
  Mux15/1 -> Deckungsschöpfung/1
  Deckungsmaterialschöpfung/1(RessourcenMengeDeckungsmaterial) -> Mux15/1
  Deckungsmaterialschöpfung/2(PreisDeckungsmaterialOut) -> Banken/8(PreisDeckungsmaterial), Mux15/2
  Deckungsmaterialschöpfung/3(AngebotsMengeDeckungsmaterial) -> Banken/9(MengeDeckungsmaterial), Mux15/3
  Deckungsmaterialschöpfung/4(Ressourcenabbaumenge) -> Mux15/4
  Banken/21(NachfrageDeckungsmaterial) -> Nachfrage Deckungsmaterial: 0/1
  Nachfrage Deckungsmaterial: 0/1 -> Deckungsmaterialschöpfung/1(NachfrageDeckungsmaterial)
  Constant: 0/1 -> Notenbankzinsatz/1
  Banken/22(Maximale Kreditvergabe) -> Maximale Geldmenge/1
